simulink model "E_8f"  (R2017a)
settings: Solver=VariableStepAuto  StartTime=0.0  StopTime=20  RelTol=1e-3
InitFcn:
  | E_param
undefined symbols (not defined in the file): E_animation, P
settings Model: Creator=Mat Haskell  LastModifiedBy=Mat Haskell

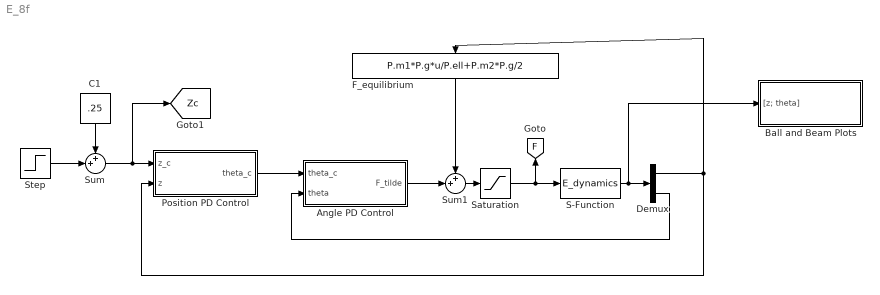
== system E_8f ==
  Angle PD Control : Subsystem
  Ball and Beam Plots : Subsystem
  C1 : Constant  Value=.25
  Demux : Demux  Outputs=2
  F_equilibrium : Fcn  Expr=P.m1*P.g*u/P.ell+P.m2*P.g/2
  Position PD Control : Subsystem
  S-Function : S-Function  FunctionName=E_dynamics  Parameters=P  SFunctionDeploymentMode=off  EnableBusSupport=off
  Saturation : Saturate  UpperLimit=15  LowerLimit=0
  Step : Step  Time=0  After=.25  SampleTime=0
  Sum : Sum  Inputs=++|
  Sum1 : Sum  Inputs=++|
  tag scope: F=global, Zc=global
  wires:
  C1/1 -> Sum/1
  Sum/1 -> [Zc], Position PD Control/1(z_c)
  S-Function/1 -> Demux/1, Ball and Beam Plots/1("[z; theta]")
  Step/1 -> Sum/2
  Position PD Control/1(theta_c) -> Angle PD Control/1(theta_c)
  Angle PD Control/1(F_tilde) -> Sum1/2
  Demux/1 -> Position PD Control/2(z), F_equilibrium/1
  Demux/2 -> Angle PD Control/2(theta)
  F_equilibrium/1 -> Sum1/1
  Sum1/1 -> Saturation/1
  Saturation/1 -> S-Function/1, [F]

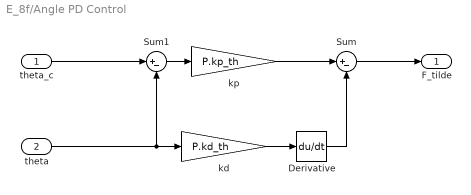
== system E_8f/Angle PD Control ==
  theta_c : Inport
  theta : Inport  Port=2
  Derivative : Derivative
  Sum : Sum  Inputs=|+-
  Sum1 : Sum  Inputs=|+-
  kd : Gain  Gain=P.kd_th
  kp : Gain  Gain=P.kp_th
  F_tilde : Outport
  wires:
  Derivative/1 -> Sum/2
  Sum1/1 -> kp/1
  theta_c/1 -> Sum1/1
  Sum/1 -> F_tilde/1
  kp/1 -> Sum/1
  kd/1 -> Derivative/1
  theta/1 -> Sum1/2, kd/1

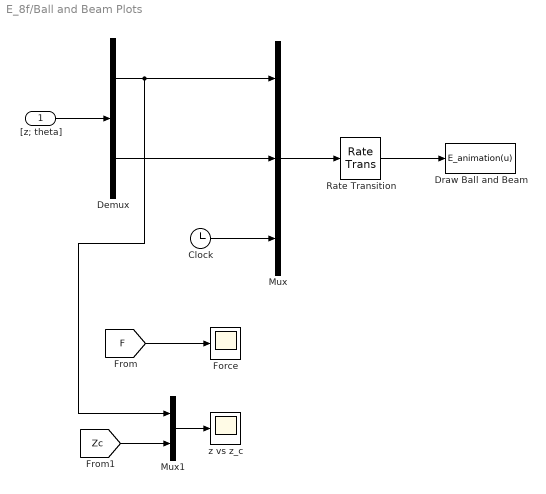
== system E_8f/Ball and Beam Plots ==
  "[z; theta]" : Inport
  Clock : Clock
  Demux : Demux  Outputs=2
  Draw Ball and Beam : MATLABFcn  MATLABFcn=E_animation(u)  OutputDimensions=0
  Force : Scope
  Mux : Mux  Inputs=3
  Mux1 : Mux  Inputs=2
  Rate Transition : RateTransition  OutPortSampleTime=P.t_plot
  z vs z_c : Scope
  wires:
  "[z; theta]"/1 -> Demux/1
  Rate Transition/1 -> Draw Ball and Beam/1
  Mux/1 -> Rate Transition/1
  Clock/1 -> Mux/3
  Demux/1 -> Mux1/1, Mux/1
  Demux/2 -> Mux/2
  [F] -> Force/1
  Mux1/1 -> z vs z_c/1
  [Zc] -> Mux1/2

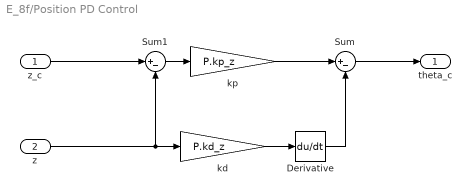
== system E_8f/Position PD Control ==
  z_c : Inport
  z : Inport  Port=2
  Derivative : Derivative
  Sum : Sum  Inputs=|+-
  Sum1 : Sum  Inputs=|+-
  kd : Gain  Gain=P.kd_z
  kp : Gain  Gain=P.kp_z
  theta_c : Outport
  wires:
  Derivative/1 -> Sum/2
  Sum1/1 -> kp/1
  z_c/1 -> Sum1/1
  Sum/1 -> theta_c/1
  kp/1 -> Sum/1
  kd/1 -> Derivative/1
  z/1 -> Sum1/2, kd/1
